simulink model "TST_InjVlv_CalcET"  (R2016b)
settings: Solver=FixedStepDiscrete  StartTime=0.0  StopTime=simTime  FixedStep=sampleTime  RelTol=1e-3
values from neighbouring files (symbols this model uses):
  testCase = 1    [initTST_InjVlv_CalcET_001.m]    (also in initTST_InjVlv_CalcET_002.m = 2)
libraries: simulink x21, UnitTest_Lib x18
settings Model: Creator=zhengjinyan  LastModifiedBy=zhengjinyan
settings DebuggingCC: SignalRangeChecking=error

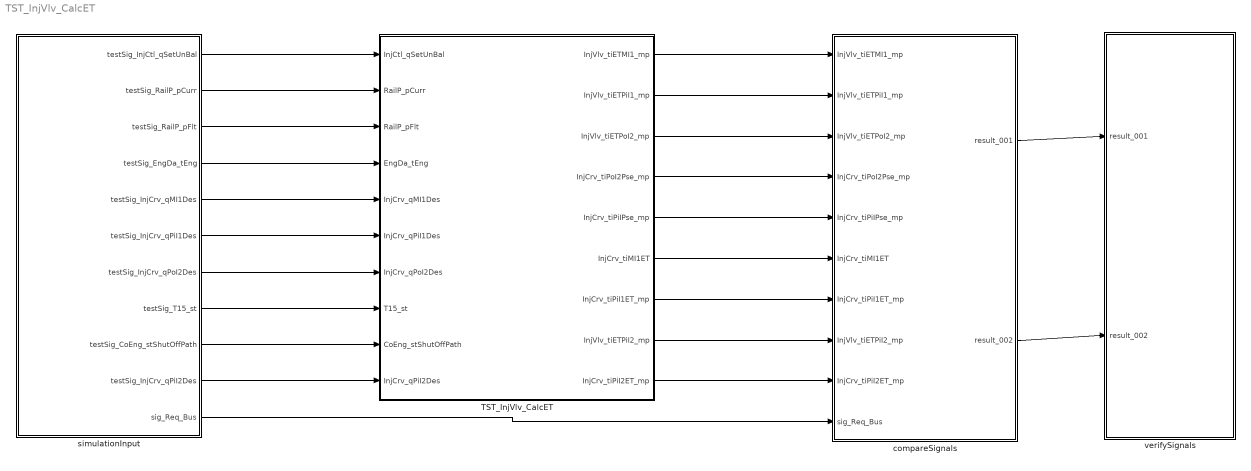
== system TST_InjVlv_CalcET ==
  TST_InjVlv_CalcET : Subsystem
  compareSignals : Subsystem
  simulationInput : Subsystem
  verifySignals : Subsystem
  wires:
  simulationInput/1(testSig_InjCtl_qSetUnBal) -> TST_InjVlv_CalcET/1(InjCtl_qSetUnBal)
  simulationInput/2(testSig_RailP_pCurr) -> TST_InjVlv_CalcET/2(RailP_pCurr)
  simulationInput/3(testSig_RailP_pFlt) -> TST_InjVlv_CalcET/3(RailP_pFlt)
  simulationInput/4(testSig_EngDa_tEng) -> TST_InjVlv_CalcET/4(EngDa_tEng)
  simulationInput/5(testSig_InjCrv_qMI1Des) -> TST_InjVlv_CalcET/5(InjCrv_qMI1Des)
  simulationInput/6(testSig_InjCrv_qPiI1Des) -> TST_InjVlv_CalcET/6(InjCrv_qPiI1Des)
  simulationInput/7(testSig_InjCrv_qPoI2Des) -> TST_InjVlv_CalcET/7(InjCrv_qPoI2Des)
  simulationInput/8(testSig_T15_st) -> TST_InjVlv_CalcET/8(T15_st)
  simulationInput/9(testSig_CoEng_stShutOffPath) -> TST_InjVlv_CalcET/9(CoEng_stShutOffPath)
  simulationInput/10(testSig_InjCrv_qPiI2Des) -> TST_InjVlv_CalcET/10(InjCrv_qPiI2Des)
  TST_InjVlv_CalcET/1(InjVlv_tiETMI1_mp) -> compareSignals/1(InjVlv_tiETMI1_mp)
  TST_InjVlv_CalcET/2(InjVlv_tiETPiI1_mp) -> compareSignals/2(InjVlv_tiETPiI1_mp)
  TST_InjVlv_CalcET/3(InjVlv_tiETPoI2_mp) -> compareSignals/3(InjVlv_tiETPoI2_mp)
  TST_InjVlv_CalcET/4(InjCrv_tiPoI2Pse_mp) -> compareSignals/4(InjCrv_tiPoI2Pse_mp)
  TST_InjVlv_CalcET/5(InjCrv_tiPiIPse_mp) -> compareSignals/5(InjCrv_tiPiIPse_mp)
  TST_InjVlv_CalcET/6(InjCrv_tiMI1ET) -> compareSignals/6(InjCrv_tiMI1ET)
  TST_InjVlv_CalcET/7(InjCrv_tiPiI1ET_mp) -> compareSignals/7(InjCrv_tiPiI1ET_mp)
  TST_InjVlv_CalcET/8(InjVlv_tiETPiI2_mp) -> compareSignals/8(InjVlv_tiETPiI2_mp)
  TST_InjVlv_CalcET/9(InjCrv_tiPiI2ET_mp) -> compareSignals/9(InjCrv_tiPiI2ET_mp)
  simulationInput/11(sig_Req_Bus) -> compareSignals/10(sig_Req_Bus)
  compareSignals/1(result_001) -> verifySignals/1(result_001)
  compareSignals/2(result_002) -> verifySignals/2(result_002)

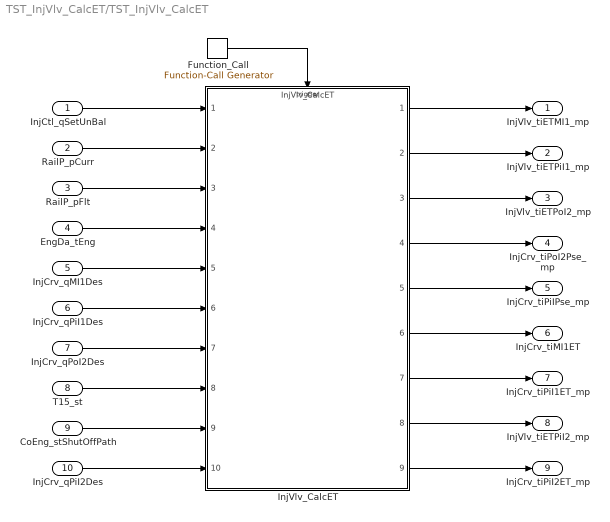
== system TST_InjVlv_CalcET/TST_InjVlv_CalcET ==
  InjCtl_qSetUnBal : Inport
  RailP_pCurr : Inport  Port=2
  RailP_pFlt : Inport  Port=3
  EngDa_tEng : Inport  Port=4
  InjCrv_qMI1Des : Inport  Port=5
  InjCrv_qPiI1Des : Inport  Port=6
  InjCrv_qPoI2Des : Inport  Port=7
  T15_st : Inport  Port=8
  CoEng_stShutOffPath : Inport  Port=9
  InjCrv_qPiI2Des : Inport  Port=10
  Function_Call : simulink/Ports & Subsystems/Function-Call Generator  sample_time=sampleTime  numberOfIterations=1
  InjVlv_CalcET : ModelReference  ModelNameDialog=InjVlv_CalcET  SimulationMode=Normal  ModelReferenceVersion=1.43  TriggerPortName=function  TriggerPortTriggerType=function-call  TriggerPortStatesWhenEnabling=held
  InjVlv_tiETMI1_mp : Outport
  InjVlv_tiETPiI1_mp : Outport  Port=2
  InjVlv_tiETPoI2_mp : Outport  Port=3
  InjCrv_tiPoI2Pse_mp : Outport  Port=4
  InjCrv_tiPiIPse_mp : Outport  Port=5
  InjCrv_tiMI1ET : Outport  Port=6
  InjCrv_tiPiI1ET_mp : Outport  Port=7
  InjVlv_tiETPiI2_mp : Outport  Port=8
  InjCrv_tiPiI2ET_mp : Outport  Port=9
  wires:
  Function_Call/1 -> InjVlv_CalcET/Trigger
  InjCtl_qSetUnBal/1 -> InjVlv_CalcET/1
  RailP_pCurr/1 -> InjVlv_CalcET/2
  RailP_pFlt/1 -> InjVlv_CalcET/3
  EngDa_tEng/1 -> InjVlv_CalcET/4
  InjCrv_qMI1Des/1 -> InjVlv_CalcET/5
  InjCrv_qPiI1Des/1 -> InjVlv_CalcET/6
  InjCrv_qPoI2Des/1 -> InjVlv_CalcET/7
  T15_st/1 -> InjVlv_CalcET/8
  CoEng_stShutOffPath/1 -> InjVlv_CalcET/9
  InjCrv_qPiI2Des/1 -> InjVlv_CalcET/10
  InjVlv_CalcET/1 -> InjVlv_tiETMI1_mp/1
  InjVlv_CalcET/2 -> InjVlv_tiETPiI1_mp/1
  InjVlv_CalcET/3 -> InjVlv_tiETPoI2_mp/1
  InjVlv_CalcET/4 -> InjCrv_tiPoI2Pse_mp/1
  InjVlv_CalcET/5 -> InjCrv_tiPiIPse_mp/1
  InjVlv_CalcET/6 -> InjCrv_tiMI1ET/1
  InjVlv_CalcET/7 -> InjCrv_tiPiI1ET_mp/1
  InjVlv_CalcET/8 -> InjVlv_tiETPiI2_mp/1
  InjVlv_CalcET/9 -> InjCrv_tiPiI2ET_mp/1

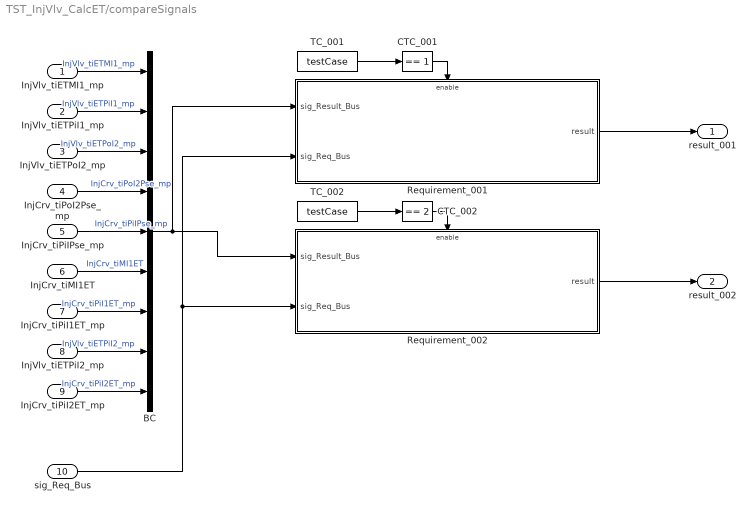
== system TST_InjVlv_CalcET/compareSignals ==
  InjVlv_tiETMI1_mp : Inport
  InjVlv_tiETPiI1_mp : Inport  Port=2
  InjVlv_tiETPoI2_mp : Inport  Port=3
  InjCrv_tiPoI2Pse_mp : Inport  Port=4
  InjCrv_tiPiIPse_mp : Inport  Port=5
  InjCrv_tiMI1ET : Inport  Port=6
  InjCrv_tiPiI1ET_mp : Inport  Port=7
  InjVlv_tiETPiI2_mp : Inport  Port=8
  InjCrv_tiPiI2ET_mp : Inport  Port=9
  sig_Req_Bus : Inport  Port=10
  BC : BusCreator  Inputs=9
  CTC_001 : simulink/Logic and Bit Operations/Compare To Constant  relop===  const=1  OutDataTypeStr=boolean
  CTC_002 : simulink/Logic and Bit Operations/Compare To Constant  relop===  const=2  OutDataTypeStr=boolean
  Requirement_001 : Subsystem
  Requirement_002 : Subsystem
  TC_001 : Constant  Value=testCase
  TC_002 : Constant  Value=testCase
  result_001 : Outport
  result_002 : Outport  Port=2
  wires:
  InjVlv_tiETMI1_mp/1 -> BC/1  "InjVlv_tiETMI1_mp"
  InjVlv_tiETPiI1_mp/1 -> BC/2  "InjVlv_tiETPiI1_mp"
  InjVlv_tiETPoI2_mp/1 -> BC/3  "InjVlv_tiETPoI2_mp"
  InjCrv_tiPoI2Pse_mp/1 -> BC/4  "InjCrv_tiPoI2Pse_mp"
  InjCrv_tiPiIPse_mp/1 -> BC/5  "InjCrv_tiPiIPse_mp"
  InjCrv_tiMI1ET/1 -> BC/6  "InjCrv_tiMI1ET"
  InjCrv_tiPiI1ET_mp/1 -> BC/7  "InjCrv_tiPiI1ET_mp"
  InjVlv_tiETPiI2_mp/1 -> BC/8  "InjVlv_tiETPiI2_mp"
  InjCrv_tiPiI2ET_mp/1 -> BC/9  "InjCrv_tiPiI2ET_mp"
  TC_001/1 -> CTC_001/1
  CTC_001/1 -> Requirement_001/Enable
  sig_Req_Bus/1 -> Requirement_001/2(sig_Req_Bus), Requirement_002/2(sig_Req_Bus)
  BC/1 -> Requirement_001/1(sig_Result_Bus), Requirement_002/1(sig_Result_Bus)
  Requirement_001/1(result) -> result_001/1
  TC_002/1 -> CTC_002/1
  CTC_002/1 -> Requirement_002/Enable
  Requirement_002/1(result) -> result_002/1

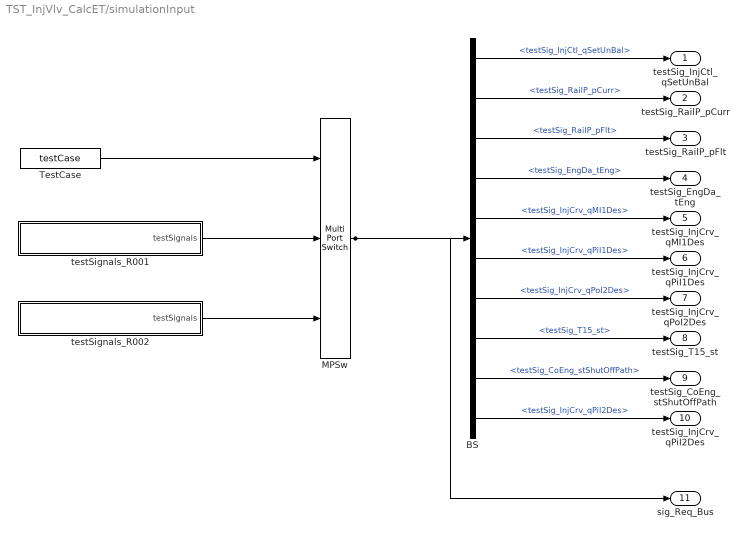
== system TST_InjVlv_CalcET/simulationInput ==
  BS : BusSelector  OutputSignals=testSig_InjCtl_qSetUnBal,testSig_RailP_pCurr,testSig_RailP_pFlt,testSig_EngDa_tEng,testSig_InjCrv_qMI1Des,testSig_InjCrv_qPiI1Des,testSig_InjCrv_qPoI2Des,testSig_T15_st,testSig_CoEng_stShutOffPath,testSig_InjCrv_qPiI2Des
  MPSw : MultiPortSwitch  Inputs=2  SaturateOnIntegerOverflow=on  InputSameDT=on
  TestCase : Constant  Value=testCase
  testSignals_R001 : Subsystem
  testSignals_R002 : Subsystem
  testSig_InjCtl_qSetUnBal : Outport
  testSig_RailP_pCurr : Outport  Port=2
  testSig_RailP_pFlt : Outport  Port=3
  testSig_EngDa_tEng : Outport  Port=4
  testSig_InjCrv_qMI1Des : Outport  Port=5
  testSig_InjCrv_qPiI1Des : Outport  Port=6
  testSig_InjCrv_qPoI2Des : Outport  Port=7
  testSig_T15_st : Outport  Port=8
  testSig_CoEng_stShutOffPath : Outport  Port=9
  testSig_InjCrv_qPiI2Des : Outport  Port=10
  sig_Req_Bus : Outport  Port=11
  wires:
  BS/1 -> testSig_InjCtl_qSetUnBal/1  "<testSig_InjCtl_qSetUnBal>"
  BS/2 -> testSig_RailP_pCurr/1  "<testSig_RailP_pCurr>"
  BS/3 -> testSig_RailP_pFlt/1  "<testSig_RailP_pFlt>"
  BS/4 -> testSig_EngDa_tEng/1  "<testSig_EngDa_tEng>"
  BS/5 -> testSig_InjCrv_qMI1Des/1  "<testSig_InjCrv_qMI1Des>"
  BS/6 -> testSig_InjCrv_qPiI1Des/1  "<testSig_InjCrv_qPiI1Des>"
  BS/7 -> testSig_InjCrv_qPoI2Des/1  "<testSig_InjCrv_qPoI2Des>"
  BS/8 -> testSig_T15_st/1  "<testSig_T15_st>"
  BS/9 -> testSig_CoEng_stShutOffPath/1  "<testSig_CoEng_stShutOffPath>"
  BS/10 -> testSig_InjCrv_qPiI2Des/1  "<testSig_InjCrv_qPiI2Des>"
  MPSw/1 -> BS/1, sig_Req_Bus/1
  TestCase/1 -> MPSw/1
  testSignals_R001/1(testSignals) -> MPSw/2
  testSignals_R002/1(testSignals) -> MPSw/3

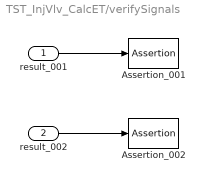
== system TST_InjVlv_CalcET/verifySignals ==
  result_001 : Inport
  result_002 : Inport  Port=2
  Assertion_001 : Assertion  Enabled=off
  Assertion_002 : Assertion  Enabled=off
  wires:
  result_001/1 -> Assertion_001/1
  result_002/1 -> Assertion_002/1

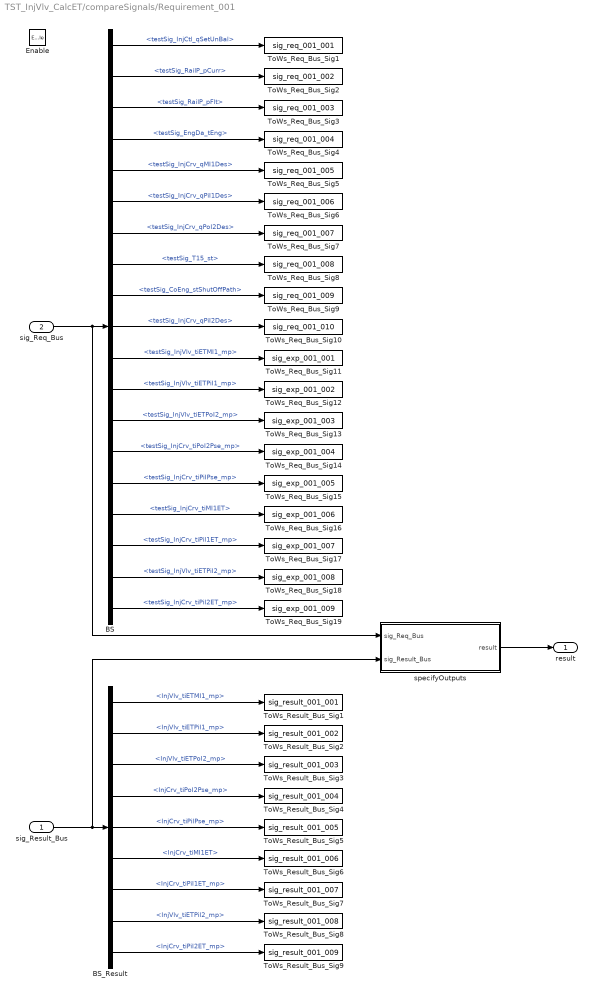
== system TST_InjVlv_CalcET/compareSignals/Requirement_001 ==
  sig_Result_Bus : Inport
  sig_Req_Bus : Inport  Port=2
  Enable : EnablePort
  BS : BusSelector  OutputSignals=testSig_InjCtl_qSetUnBal,testSig_RailP_pCurr,testSig_RailP_pFlt,testSig_EngDa_tEng,testSig_InjCrv_qMI1Des,testSig_InjCrv_qPiI1Des,testSig_InjCrv_qPoI2Des,testSig_T15_st,testSig_CoEng_stShutOffPath,testSig_InjCrv_qPiI2Des,testSig_InjVlv_tiETMI1_mp,testSig_InjVlv_tiETPiI1_mp,testSig_InjVlv_tiETPoI2_mp,testSig_InjCrv_tiPoI2Pse_mp,testSig_InjCrv_tiPiIPse_mp,testSig_InjCrv_tiMI1ET,testSig_InjCrv_tiPiI1ET_mp,testSig_InjVlv_tiETPiI2_mp,testSig_InjCrv_tiPiI2ET_mp
  BS_Result : BusSelector  OutputSignals=InjVlv_tiETMI1_mp,InjVlv_tiETPiI1_mp,InjVlv_tiETPoI2_mp,InjCrv_tiPoI2Pse_mp,InjCrv_tiPiIPse_mp,InjCrv_tiMI1ET,InjCrv_tiPiI1ET_mp,InjVlv_tiETPiI2_mp,InjCrv_tiPiI2ET_mp
  ToWs_Req_Bus_Sig1 : ToWorkspace  VariableName=sig_req_001_001  SaveFormat=Structure With Time
  ToWs_Req_Bus_Sig10 : ToWorkspace  VariableName=sig_req_001_010  SaveFormat=Structure With Time
  ToWs_Req_Bus_Sig11 : ToWorkspace  VariableName=sig_exp_001_001  SaveFormat=Structure With Time
  ToWs_Req_Bus_Sig12 : ToWorkspace  VariableName=sig_exp_001_002  SaveFormat=Structure With Time
  ToWs_Req_Bus_Sig13 : ToWorkspace  VariableName=sig_exp_001_003  SaveFormat=Structure With Time
  ToWs_Req_Bus_Sig14 : ToWorkspace  VariableName=sig_exp_001_004  SaveFormat=Structure With Time
  ToWs_Req_Bus_Sig15 : ToWorkspace  VariableName=sig_exp_001_005  SaveFormat=Structure With Time
  ToWs_Req_Bus_Sig16 : ToWorkspace  VariableName=sig_exp_001_006  SaveFormat=Structure With Time
  ToWs_Req_Bus_Sig17 : ToWorkspace  VariableName=sig_exp_001_007  SaveFormat=Structure With Time
  ToWs_Req_Bus_Sig18 : ToWorkspace  VariableName=sig_exp_001_008  SaveFormat=Structure With Time
  ToWs_Req_Bus_Sig19 : ToWorkspace  VariableName=sig_exp_001_009  SaveFormat=Structure With Time
  ToWs_Req_Bus_Sig2 : ToWorkspace  VariableName=sig_req_001_002  SaveFormat=Structure With Time
  ToWs_Req_Bus_Sig3 : ToWorkspace  VariableName=sig_req_001_003  SaveFormat=Structure With Time
  ToWs_Req_Bus_Sig4 : ToWorkspace  VariableName=sig_req_001_004  SaveFormat=Structure With Time
  ToWs_Req_Bus_Sig5 : ToWorkspace  VariableName=sig_req_001_005  SaveFormat=Structure With Time
  ToWs_Req_Bus_Sig6 : ToWorkspace  VariableName=sig_req_001_006  SaveFormat=Structure With Time
  ToWs_Req_Bus_Sig7 : ToWorkspace  VariableName=sig_req_001_007  SaveFormat=Structure With Time
  ToWs_Req_Bus_Sig8 : ToWorkspace  VariableName=sig_req_001_008  SaveFormat=Structure With Time
  ToWs_Req_Bus_Sig9 : ToWorkspace  VariableName=sig_req_001_009  SaveFormat=Structure With Time
  ToWs_Result_Bus_Sig1 : ToWorkspace  VariableName=sig_result_001_001  SaveFormat=Structure With Time
  ToWs_Result_Bus_Sig2 : ToWorkspace  VariableName=sig_result_001_002  SaveFormat=Structure With Time
  ToWs_Result_Bus_Sig3 : ToWorkspace  VariableName=sig_result_001_003  SaveFormat=Structure With Time
  ToWs_Result_Bus_Sig4 : ToWorkspace  VariableName=sig_result_001_004  SaveFormat=Structure With Time
  ToWs_Result_Bus_Sig5 : ToWorkspace  VariableName=sig_result_001_005  SaveFormat=Structure With Time
  ToWs_Result_Bus_Sig6 : ToWorkspace  VariableName=sig_result_001_006  SaveFormat=Structure With Time
  ToWs_Result_Bus_Sig7 : ToWorkspace  VariableName=sig_result_001_007  SaveFormat=Structure With Time
  ToWs_Result_Bus_Sig8 : ToWorkspace  VariableName=sig_result_001_008  SaveFormat=Structure With Time
  ToWs_Result_Bus_Sig9 : ToWorkspace  VariableName=sig_result_001_009  SaveFormat=Structure With Time
  specifyOutputs : Subsystem
  result : Outport
  wires:
  sig_Req_Bus/1 -> BS/1, specifyOutputs/1(sig_Req_Bus)
  BS/1 -> ToWs_Req_Bus_Sig1/1  "<testSig_InjCtl_qSetUnBal>"
  BS/2 -> ToWs_Req_Bus_Sig2/1  "<testSig_RailP_pCurr>"
  BS/3 -> ToWs_Req_Bus_Sig3/1  "<testSig_RailP_pFlt>"
  BS/4 -> ToWs_Req_Bus_Sig4/1  "<testSig_EngDa_tEng>"
  BS/5 -> ToWs_Req_Bus_Sig5/1  "<testSig_InjCrv_qMI1Des>"
  BS/6 -> ToWs_Req_Bus_Sig6/1  "<testSig_InjCrv_qPiI1Des>"
  BS/7 -> ToWs_Req_Bus_Sig7/1  "<testSig_InjCrv_qPoI2Des>"
  BS/8 -> ToWs_Req_Bus_Sig8/1  "<testSig_T15_st>"
  BS/9 -> ToWs_Req_Bus_Sig9/1  "<testSig_CoEng_stShutOffPath>"
  BS/10 -> ToWs_Req_Bus_Sig10/1  "<testSig_InjCrv_qPiI2Des>"
  BS/11 -> ToWs_Req_Bus_Sig11/1  "<testSig_InjVlv_tiETMI1_mp>"
  BS/12 -> ToWs_Req_Bus_Sig12/1  "<testSig_InjVlv_tiETPiI1_mp>"
  BS/13 -> ToWs_Req_Bus_Sig13/1  "<testSig_InjVlv_tiETPoI2_mp>"
  BS/14 -> ToWs_Req_Bus_Sig14/1  "<testSig_InjCrv_tiPoI2Pse_mp>"
  BS/15 -> ToWs_Req_Bus_Sig15/1  "<testSig_InjCrv_tiPiIPse_mp>"
  BS/16 -> ToWs_Req_Bus_Sig16/1  "<testSig_InjCrv_tiMI1ET>"
  BS/17 -> ToWs_Req_Bus_Sig17/1  "<testSig_InjCrv_tiPiI1ET_mp>"
  BS/18 -> ToWs_Req_Bus_Sig18/1  "<testSig_InjVlv_tiETPiI2_mp>"
  BS/19 -> ToWs_Req_Bus_Sig19/1  "<testSig_InjCrv_tiPiI2ET_mp>"
  sig_Result_Bus/1 -> BS_Result/1, specifyOutputs/2(sig_Result_Bus)
  BS_Result/1 -> ToWs_Result_Bus_Sig1/1  "<InjVlv_tiETMI1_mp>"
  BS_Result/2 -> ToWs_Result_Bus_Sig2/1  "<InjVlv_tiETPiI1_mp>"
  BS_Result/3 -> ToWs_Result_Bus_Sig3/1  "<InjVlv_tiETPoI2_mp>"
  BS_Result/4 -> ToWs_Result_Bus_Sig4/1  "<InjCrv_tiPoI2Pse_mp>"
  BS_Result/5 -> ToWs_Result_Bus_Sig5/1  "<InjCrv_tiPiIPse_mp>"
  BS_Result/6 -> ToWs_Result_Bus_Sig6/1  "<InjCrv_tiMI1ET>"
  BS_Result/7 -> ToWs_Result_Bus_Sig7/1  "<InjCrv_tiPiI1ET_mp>"
  BS_Result/8 -> ToWs_Result_Bus_Sig8/1  "<InjVlv_tiETPiI2_mp>"
  BS_Result/9 -> ToWs_Result_Bus_Sig9/1  "<InjCrv_tiPiI2ET_mp>"
  specifyOutputs/1(result) -> result/1

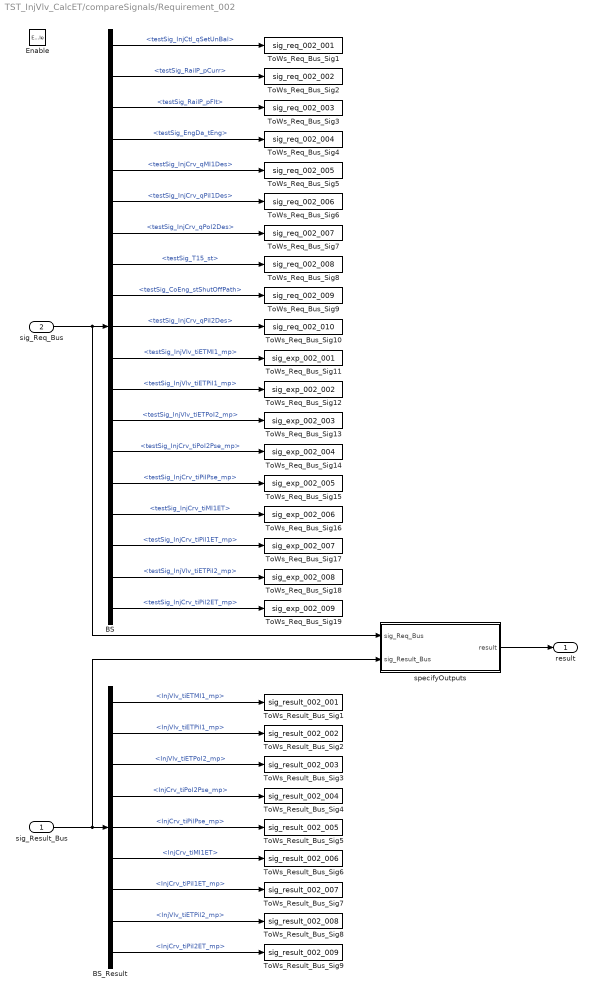
== system TST_InjVlv_CalcET/compareSignals/Requirement_002 ==
  sig_Result_Bus : Inport
  sig_Req_Bus : Inport  Port=2
  Enable : EnablePort
  BS : BusSelector  OutputSignals=testSig_InjCtl_qSetUnBal,testSig_RailP_pCurr,testSig_RailP_pFlt,testSig_EngDa_tEng,testSig_InjCrv_qMI1Des,testSig_InjCrv_qPiI1Des,testSig_InjCrv_qPoI2Des,testSig_T15_st,testSig_CoEng_stShutOffPath,testSig_InjCrv_qPiI2Des,testSig_InjVlv_tiETMI1_mp,testSig_InjVlv_tiETPiI1_mp,testSig_InjVlv_tiETPoI2_mp,testSig_InjCrv_tiPoI2Pse_mp,testSig_InjCrv_tiPiIPse_mp,testSig_InjCrv_tiMI1ET,testSig_InjCrv_tiPiI1ET_mp,testSig_InjVlv_tiETPiI2_mp,testSig_InjCrv_tiPiI2ET_mp
  BS_Result : BusSelector  OutputSignals=InjVlv_tiETMI1_mp,InjVlv_tiETPiI1_mp,InjVlv_tiETPoI2_mp,InjCrv_tiPoI2Pse_mp,InjCrv_tiPiIPse_mp,InjCrv_tiMI1ET,InjCrv_tiPiI1ET_mp,InjVlv_tiETPiI2_mp,InjCrv_tiPiI2ET_mp
  ToWs_Req_Bus_Sig1 : ToWorkspace  VariableName=sig_req_002_001  SaveFormat=Structure With Time
  ToWs_Req_Bus_Sig10 : ToWorkspace  VariableName=sig_req_002_010  SaveFormat=Structure With Time
  ToWs_Req_Bus_Sig11 : ToWorkspace  VariableName=sig_exp_002_001  SaveFormat=Structure With Time
  ToWs_Req_Bus_Sig12 : ToWorkspace  VariableName=sig_exp_002_002  SaveFormat=Structure With Time
  ToWs_Req_Bus_Sig13 : ToWorkspace  VariableName=sig_exp_002_003  SaveFormat=Structure With Time
  ToWs_Req_Bus_Sig14 : ToWorkspace  VariableName=sig_exp_002_004  SaveFormat=Structure With Time
  ToWs_Req_Bus_Sig15 : ToWorkspace  VariableName=sig_exp_002_005  SaveFormat=Structure With Time
  ToWs_Req_Bus_Sig16 : ToWorkspace  VariableName=sig_exp_002_006  SaveFormat=Structure With Time
  ToWs_Req_Bus_Sig17 : ToWorkspace  VariableName=sig_exp_002_007  SaveFormat=Structure With Time
  ToWs_Req_Bus_Sig18 : ToWorkspace  VariableName=sig_exp_002_008  SaveFormat=Structure With Time
  ToWs_Req_Bus_Sig19 : ToWorkspace  VariableName=sig_exp_002_009  SaveFormat=Structure With Time
  ToWs_Req_Bus_Sig2 : ToWorkspace  VariableName=sig_req_002_002  SaveFormat=Structure With Time
  ToWs_Req_Bus_Sig3 : ToWorkspace  VariableName=sig_req_002_003  SaveFormat=Structure With Time
  ToWs_Req_Bus_Sig4 : ToWorkspace  VariableName=sig_req_002_004  SaveFormat=Structure With Time
  ToWs_Req_Bus_Sig5 : ToWorkspace  VariableName=sig_req_002_005  SaveFormat=Structure With Time
  ToWs_Req_Bus_Sig6 : ToWorkspace  VariableName=sig_req_002_006  SaveFormat=Structure With Time
  ToWs_Req_Bus_Sig7 : ToWorkspace  VariableName=sig_req_002_007  SaveFormat=Structure With Time
  ToWs_Req_Bus_Sig8 : ToWorkspace  VariableName=sig_req_002_008  SaveFormat=Structure With Time
  ToWs_Req_Bus_Sig9 : ToWorkspace  VariableName=sig_req_002_009  SaveFormat=Structure With Time
  ToWs_Result_Bus_Sig1 : ToWorkspace  VariableName=sig_result_002_001  SaveFormat=Structure With Time
  ToWs_Result_Bus_Sig2 : ToWorkspace  VariableName=sig_result_002_002  SaveFormat=Structure With Time
  ToWs_Result_Bus_Sig3 : ToWorkspace  VariableName=sig_result_002_003  SaveFormat=Structure With Time
  ToWs_Result_Bus_Sig4 : ToWorkspace  VariableName=sig_result_002_004  SaveFormat=Structure With Time
  ToWs_Result_Bus_Sig5 : ToWorkspace  VariableName=sig_result_002_005  SaveFormat=Structure With Time
  ToWs_Result_Bus_Sig6 : ToWorkspace  VariableName=sig_result_002_006  SaveFormat=Structure With Time
  ToWs_Result_Bus_Sig7 : ToWorkspace  VariableName=sig_result_002_007  SaveFormat=Structure With Time
  ToWs_Result_Bus_Sig8 : ToWorkspace  VariableName=sig_result_002_008  SaveFormat=Structure With Time
  ToWs_Result_Bus_Sig9 : ToWorkspace  VariableName=sig_result_002_009  SaveFormat=Structure With Time
  specifyOutputs : Subsystem
  result : Outport
  wires:
  sig_Req_Bus/1 -> BS/1, specifyOutputs/1(sig_Req_Bus)
  BS/1 -> ToWs_Req_Bus_Sig1/1  "<testSig_InjCtl_qSetUnBal>"
  BS/2 -> ToWs_Req_Bus_Sig2/1  "<testSig_RailP_pCurr>"
  BS/3 -> ToWs_Req_Bus_Sig3/1  "<testSig_RailP_pFlt>"
  BS/4 -> ToWs_Req_Bus_Sig4/1  "<testSig_EngDa_tEng>"
  BS/5 -> ToWs_Req_Bus_Sig5/1  "<testSig_InjCrv_qMI1Des>"
  BS/6 -> ToWs_Req_Bus_Sig6/1  "<testSig_InjCrv_qPiI1Des>"
  BS/7 -> ToWs_Req_Bus_Sig7/1  "<testSig_InjCrv_qPoI2Des>"
  BS/8 -> ToWs_Req_Bus_Sig8/1  "<testSig_T15_st>"
  BS/9 -> ToWs_Req_Bus_Sig9/1  "<testSig_CoEng_stShutOffPath>"
  BS/10 -> ToWs_Req_Bus_Sig10/1  "<testSig_InjCrv_qPiI2Des>"
  BS/11 -> ToWs_Req_Bus_Sig11/1  "<testSig_InjVlv_tiETMI1_mp>"
  BS/12 -> ToWs_Req_Bus_Sig12/1  "<testSig_InjVlv_tiETPiI1_mp>"
  BS/13 -> ToWs_Req_Bus_Sig13/1  "<testSig_InjVlv_tiETPoI2_mp>"
  BS/14 -> ToWs_Req_Bus_Sig14/1  "<testSig_InjCrv_tiPoI2Pse_mp>"
  BS/15 -> ToWs_Req_Bus_Sig15/1  "<testSig_InjCrv_tiPiIPse_mp>"
  BS/16 -> ToWs_Req_Bus_Sig16/1  "<testSig_InjCrv_tiMI1ET>"
  BS/17 -> ToWs_Req_Bus_Sig17/1  "<testSig_InjCrv_tiPiI1ET_mp>"
  BS/18 -> ToWs_Req_Bus_Sig18/1  "<testSig_InjVlv_tiETPiI2_mp>"
  BS/19 -> ToWs_Req_Bus_Sig19/1  "<testSig_InjCrv_tiPiI2ET_mp>"
  sig_Result_Bus/1 -> BS_Result/1, specifyOutputs/2(sig_Result_Bus)
  BS_Result/1 -> ToWs_Result_Bus_Sig1/1  "<InjVlv_tiETMI1_mp>"
  BS_Result/2 -> ToWs_Result_Bus_Sig2/1  "<InjVlv_tiETPiI1_mp>"
  BS_Result/3 -> ToWs_Result_Bus_Sig3/1  "<InjVlv_tiETPoI2_mp>"
  BS_Result/4 -> ToWs_Result_Bus_Sig4/1  "<InjCrv_tiPoI2Pse_mp>"
  BS_Result/5 -> ToWs_Result_Bus_Sig5/1  "<InjCrv_tiPiIPse_mp>"
  BS_Result/6 -> ToWs_Result_Bus_Sig6/1  "<InjCrv_tiMI1ET>"
  BS_Result/7 -> ToWs_Result_Bus_Sig7/1  "<InjCrv_tiPiI1ET_mp>"
  BS_Result/8 -> ToWs_Result_Bus_Sig8/1  "<InjVlv_tiETPiI2_mp>"
  BS_Result/9 -> ToWs_Result_Bus_Sig9/1  "<InjCrv_tiPiI2ET_mp>"
  specifyOutputs/1(result) -> result/1

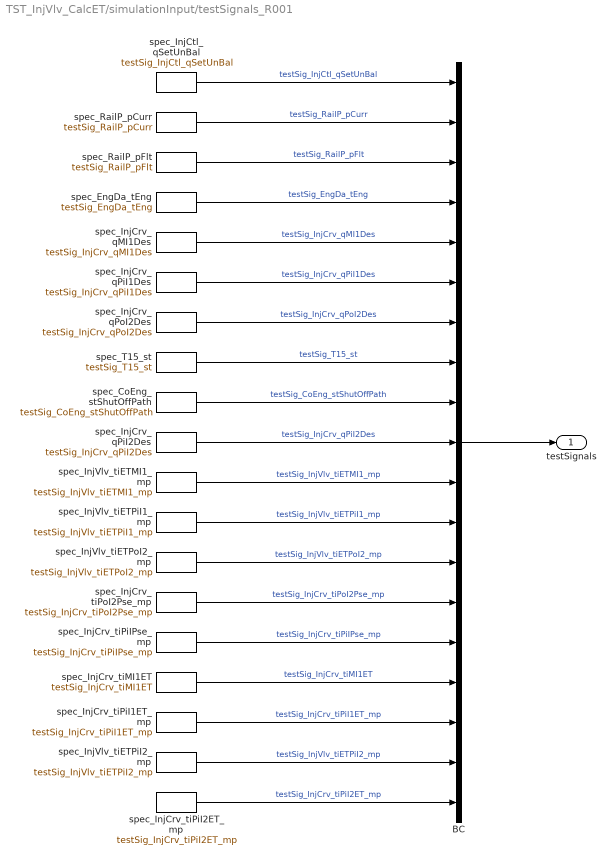
== system TST_InjVlv_CalcET/simulationInput/testSignals_R001 ==
  BC : BusCreator  Inputs=19
  spec_CoEng_stShutOffPath : FromWorkspace  VariableName=testSig_CoEng_stShutOffPath  Interpolate=off  OutputAfterFinalValue=Holding final value
  spec_EngDa_tEng : FromWorkspace  VariableName=testSig_EngDa_tEng  Interpolate=off  OutputAfterFinalValue=Holding final value
  spec_InjCrv_qMI1Des : FromWorkspace  VariableName=testSig_InjCrv_qMI1Des  Interpolate=off  OutputAfterFinalValue=Holding final value
  spec_InjCrv_qPiI1Des : FromWorkspace  VariableName=testSig_InjCrv_qPiI1Des  Interpolate=off  OutputAfterFinalValue=Holding final value
  spec_InjCrv_qPiI2Des : FromWorkspace  VariableName=testSig_InjCrv_qPiI2Des  Interpolate=off  OutputAfterFinalValue=Holding final value
  spec_InjCrv_qPoI2Des : FromWorkspace  VariableName=testSig_InjCrv_qPoI2Des  Interpolate=off  OutputAfterFinalValue=Holding final value
  spec_InjCrv_tiMI1ET : FromWorkspace  VariableName=testSig_InjCrv_tiMI1ET  Interpolate=off  OutputAfterFinalValue=Holding final value
  spec_InjCrv_tiPiI1ET_mp : FromWorkspace  VariableName=testSig_InjCrv_tiPiI1ET_mp  Interpolate=off  OutputAfterFinalValue=Holding final value
  spec_InjCrv_tiPiI2ET_mp : FromWorkspace  VariableName=testSig_InjCrv_tiPiI2ET_mp  Interpolate=off  OutputAfterFinalValue=Holding final value
  spec_InjCrv_tiPiIPse_mp : FromWorkspace  VariableName=testSig_InjCrv_tiPiIPse_mp  Interpolate=off  OutputAfterFinalValue=Holding final value
  spec_InjCrv_tiPoI2Pse_mp : FromWorkspace  VariableName=testSig_InjCrv_tiPoI2Pse_mp  Interpolate=off  OutputAfterFinalValue=Holding final value
  spec_InjCtl_qSetUnBal : FromWorkspace  VariableName=testSig_InjCtl_qSetUnBal  Interpolate=off  OutputAfterFinalValue=Holding final value
  spec_InjVlv_tiETMI1_mp : FromWorkspace  VariableName=testSig_InjVlv_tiETMI1_mp  Interpolate=off  OutputAfterFinalValue=Holding final value
  spec_InjVlv_tiETPiI1_mp : FromWorkspace  VariableName=testSig_InjVlv_tiETPiI1_mp  Interpolate=off  OutputAfterFinalValue=Holding final value
  spec_InjVlv_tiETPiI2_mp : FromWorkspace  VariableName=testSig_InjVlv_tiETPiI2_mp  Interpolate=off  OutputAfterFinalValue=Holding final value
  spec_InjVlv_tiETPoI2_mp : FromWorkspace  VariableName=testSig_InjVlv_tiETPoI2_mp  Interpolate=off  OutputAfterFinalValue=Holding final value
  spec_RailP_pCurr : FromWorkspace  VariableName=testSig_RailP_pCurr  Interpolate=off  OutputAfterFinalValue=Holding final value
  spec_RailP_pFlt : FromWorkspace  VariableName=testSig_RailP_pFlt  Interpolate=off  OutputAfterFinalValue=Holding final value
  spec_T15_st : FromWorkspace  VariableName=testSig_T15_st  Interpolate=off  OutputAfterFinalValue=Holding final value
  testSignals : Outport
  wires:
  BC/1 -> testSignals/1
  spec_InjCtl_qSetUnBal/1 -> BC/1  "testSig_InjCtl_qSetUnBal"
  spec_RailP_pCurr/1 -> BC/2  "testSig_RailP_pCurr"
  spec_RailP_pFlt/1 -> BC/3  "testSig_RailP_pFlt"
  spec_EngDa_tEng/1 -> BC/4  "testSig_EngDa_tEng"
  spec_InjCrv_qMI1Des/1 -> BC/5  "testSig_InjCrv_qMI1Des"
  spec_InjCrv_qPiI1Des/1 -> BC/6  "testSig_InjCrv_qPiI1Des"
  spec_InjCrv_qPoI2Des/1 -> BC/7  "testSig_InjCrv_qPoI2Des"
  spec_T15_st/1 -> BC/8  "testSig_T15_st"
  spec_CoEng_stShutOffPath/1 -> BC/9  "testSig_CoEng_stShutOffPath"
  spec_InjCrv_qPiI2Des/1 -> BC/10  "testSig_InjCrv_qPiI2Des"
  spec_InjVlv_tiETMI1_mp/1 -> BC/11  "testSig_InjVlv_tiETMI1_mp"
  spec_InjVlv_tiETPiI1_mp/1 -> BC/12  "testSig_InjVlv_tiETPiI1_mp"
  spec_InjVlv_tiETPoI2_mp/1 -> BC/13  "testSig_InjVlv_tiETPoI2_mp"
  spec_InjCrv_tiPoI2Pse_mp/1 -> BC/14  "testSig_InjCrv_tiPoI2Pse_mp"
  spec_InjCrv_tiPiIPse_mp/1 -> BC/15  "testSig_InjCrv_tiPiIPse_mp"
  spec_InjCrv_tiMI1ET/1 -> BC/16  "testSig_InjCrv_tiMI1ET"
  spec_InjCrv_tiPiI1ET_mp/1 -> BC/17  "testSig_InjCrv_tiPiI1ET_mp"
  spec_InjVlv_tiETPiI2_mp/1 -> BC/18  "testSig_InjVlv_tiETPiI2_mp"
  spec_InjCrv_tiPiI2ET_mp/1 -> BC/19  "testSig_InjCrv_tiPiI2ET_mp"

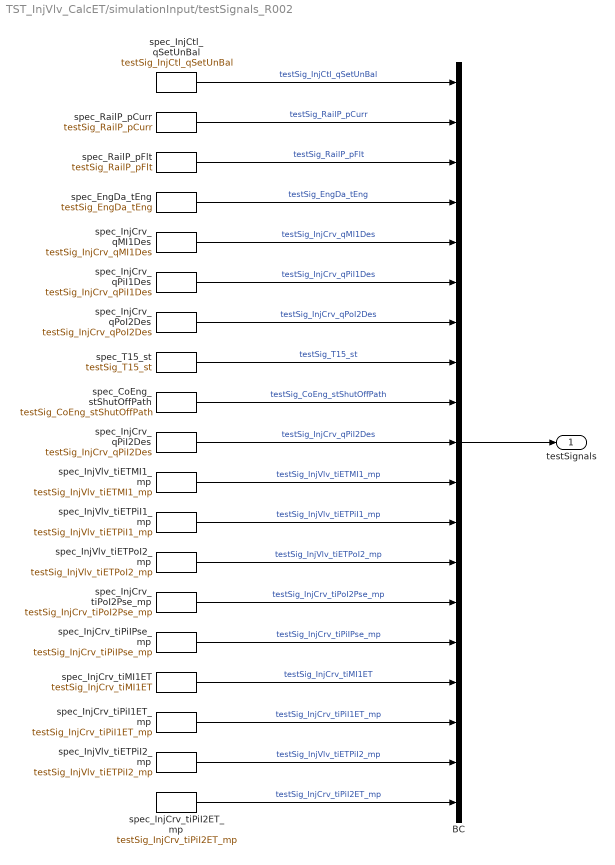
== system TST_InjVlv_CalcET/simulationInput/testSignals_R002 ==
  BC : BusCreator  Inputs=19
  spec_CoEng_stShutOffPath : FromWorkspace  VariableName=testSig_CoEng_stShutOffPath  Interpolate=off  OutputAfterFinalValue=Holding final value
  spec_EngDa_tEng : FromWorkspace  VariableName=testSig_EngDa_tEng  Interpolate=off  OutputAfterFinalValue=Holding final value
  spec_InjCrv_qMI1Des : FromWorkspace  VariableName=testSig_InjCrv_qMI1Des  Interpolate=off  OutputAfterFinalValue=Holding final value
  spec_InjCrv_qPiI1Des : FromWorkspace  VariableName=testSig_InjCrv_qPiI1Des  Interpolate=off  OutputAfterFinalValue=Holding final value
  spec_InjCrv_qPiI2Des : FromWorkspace  VariableName=testSig_InjCrv_qPiI2Des  Interpolate=off  OutputAfterFinalValue=Holding final value
  spec_InjCrv_qPoI2Des : FromWorkspace  VariableName=testSig_InjCrv_qPoI2Des  Interpolate=off  OutputAfterFinalValue=Holding final value
  spec_InjCrv_tiMI1ET : FromWorkspace  VariableName=testSig_InjCrv_tiMI1ET  Interpolate=off  OutputAfterFinalValue=Holding final value
  spec_InjCrv_tiPiI1ET_mp : FromWorkspace  VariableName=testSig_InjCrv_tiPiI1ET_mp  Interpolate=off  OutputAfterFinalValue=Holding final value
  spec_InjCrv_tiPiI2ET_mp : FromWorkspace  VariableName=testSig_InjCrv_tiPiI2ET_mp  Interpolate=off  OutputAfterFinalValue=Holding final value
  spec_InjCrv_tiPiIPse_mp : FromWorkspace  VariableName=testSig_InjCrv_tiPiIPse_mp  Interpolate=off  OutputAfterFinalValue=Holding final value
  spec_InjCrv_tiPoI2Pse_mp : FromWorkspace  VariableName=testSig_InjCrv_tiPoI2Pse_mp  Interpolate=off  OutputAfterFinalValue=Holding final value
  spec_InjCtl_qSetUnBal : FromWorkspace  VariableName=testSig_InjCtl_qSetUnBal  Interpolate=off  OutputAfterFinalValue=Holding final value
  spec_InjVlv_tiETMI1_mp : FromWorkspace  VariableName=testSig_InjVlv_tiETMI1_mp  Interpolate=off  OutputAfterFinalValue=Holding final value
  spec_InjVlv_tiETPiI1_mp : FromWorkspace  VariableName=testSig_InjVlv_tiETPiI1_mp  Interpolate=off  OutputAfterFinalValue=Holding final value
  spec_InjVlv_tiETPiI2_mp : FromWorkspace  VariableName=testSig_InjVlv_tiETPiI2_mp  Interpolate=off  OutputAfterFinalValue=Holding final value
  spec_InjVlv_tiETPoI2_mp : FromWorkspace  VariableName=testSig_InjVlv_tiETPoI2_mp  Interpolate=off  OutputAfterFinalValue=Holding final value
  spec_RailP_pCurr : FromWorkspace  VariableName=testSig_RailP_pCurr  Interpolate=off  OutputAfterFinalValue=Holding final value
  spec_RailP_pFlt : FromWorkspace  VariableName=testSig_RailP_pFlt  Interpolate=off  OutputAfterFinalValue=Holding final value
  spec_T15_st : FromWorkspace  VariableName=testSig_T15_st  Interpolate=off  OutputAfterFinalValue=Holding final value
  testSignals : Outport
  wires:
  BC/1 -> testSignals/1
  spec_InjCtl_qSetUnBal/1 -> BC/1  "testSig_InjCtl_qSetUnBal"
  spec_RailP_pCurr/1 -> BC/2  "testSig_RailP_pCurr"
  spec_RailP_pFlt/1 -> BC/3  "testSig_RailP_pFlt"
  spec_EngDa_tEng/1 -> BC/4  "testSig_EngDa_tEng"
  spec_InjCrv_qMI1Des/1 -> BC/5  "testSig_InjCrv_qMI1Des"
  spec_InjCrv_qPiI1Des/1 -> BC/6  "testSig_InjCrv_qPiI1Des"
  spec_InjCrv_qPoI2Des/1 -> BC/7  "testSig_InjCrv_qPoI2Des"
  spec_T15_st/1 -> BC/8  "testSig_T15_st"
  spec_CoEng_stShutOffPath/1 -> BC/9  "testSig_CoEng_stShutOffPath"
  spec_InjCrv_qPiI2Des/1 -> BC/10  "testSig_InjCrv_qPiI2Des"
  spec_InjVlv_tiETMI1_mp/1 -> BC/11  "testSig_InjVlv_tiETMI1_mp"
  spec_InjVlv_tiETPiI1_mp/1 -> BC/12  "testSig_InjVlv_tiETPiI1_mp"
  spec_InjVlv_tiETPoI2_mp/1 -> BC/13  "testSig_InjVlv_tiETPoI2_mp"
  spec_InjCrv_tiPoI2Pse_mp/1 -> BC/14  "testSig_InjCrv_tiPoI2Pse_mp"
  spec_InjCrv_tiPiIPse_mp/1 -> BC/15  "testSig_InjCrv_tiPiIPse_mp"
  spec_InjCrv_tiMI1ET/1 -> BC/16  "testSig_InjCrv_tiMI1ET"
  spec_InjCrv_tiPiI1ET_mp/1 -> BC/17  "testSig_InjCrv_tiPiI1ET_mp"
  spec_InjVlv_tiETPiI2_mp/1 -> BC/18  "testSig_InjVlv_tiETPiI2_mp"
  spec_InjCrv_tiPiI2ET_mp/1 -> BC/19  "testSig_InjCrv_tiPiI2ET_mp"

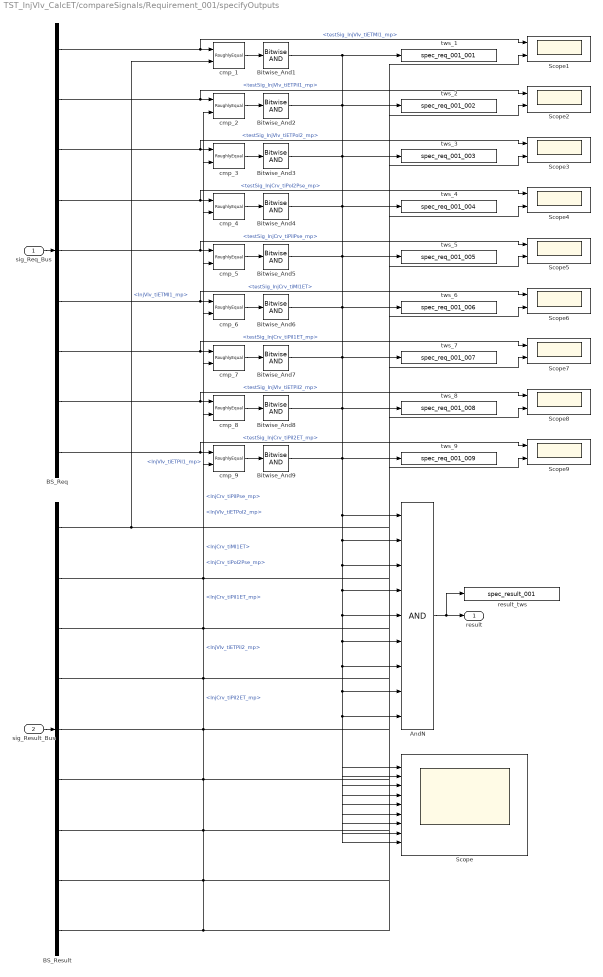
== system TST_InjVlv_CalcET/compareSignals/Requirement_001/specifyOutputs ==
  sig_Req_Bus : Inport
  sig_Result_Bus : Inport  Port=2
  AndN : Logic  Inputs=9
  BS_Req : BusSelector  OutputSignals=testSig_InjVlv_tiETMI1_mp,testSig_InjVlv_tiETPiI1_mp,testSig_InjVlv_tiETPoI2_mp,testSig_InjCrv_tiPoI2Pse_mp,testSig_InjCrv_tiPiIPse_mp,testSig_InjCrv_tiMI1ET,testSig_InjCrv_tiPiI1ET_mp,testSig_InjVlv_tiETPiI2_mp,testSig_InjCrv_tiPiI2ET_mp
  BS_Result : BusSelector  OutputSignals=InjVlv_tiETMI1_mp,InjVlv_tiETPiI1_mp,InjVlv_tiETPoI2_mp,InjCrv_tiPoI2Pse_mp,InjCrv_tiPiIPse_mp,InjCrv_tiMI1ET,InjCrv_tiPiI1ET_mp,InjVlv_tiETPiI2_mp,InjCrv_tiPiI2ET_mp
  Bitwise_And{1..9} (9 alike) : simulink/Logic and Bit Operations/Bitwise Operator  logicop=AND  UseBitMask=off  BitMask=bin2dec('11011001')  BitMaskRealWorld=Stored Integer
  Scope : Scope  NumInputPorts=9
  Scope{1..9} (9 alike) : Scope  NumInputPorts=2
  cmp_{1..9} (9 alike) : UnitTest_Lib/RoughlyEqual  slope=1
  result_tws : ToWorkspace  VariableName=spec_result_001
  tws_1 : ToWorkspace  VariableName=spec_req_001_001
  tws_2 : ToWorkspace  VariableName=spec_req_001_002
  tws_3 : ToWorkspace  VariableName=spec_req_001_003
  tws_4 : ToWorkspace  VariableName=spec_req_001_004
  tws_5 : ToWorkspace  VariableName=spec_req_001_005
  tws_6 : ToWorkspace  VariableName=spec_req_001_006
  tws_7 : ToWorkspace  VariableName=spec_req_001_007
  tws_8 : ToWorkspace  VariableName=spec_req_001_008
  tws_9 : ToWorkspace  VariableName=spec_req_001_009
  result : Outport
  wires:
  sig_Req_Bus/1 -> BS_Req/1
  sig_Result_Bus/1 -> BS_Result/1
  AndN/1 -> result/1, result_tws/1
  BS_Req/1 -> cmp_1/1, Scope1/1  "<testSig_InjVlv_tiETMI1_mp>"
  BS_Result/1 -> cmp_1/2, Scope1/2  "<InjVlv_tiETMI1_mp>"
  cmp_1/1 -> Bitwise_And1/1
  Bitwise_And1/1 -> AndN/1, Scope/1, tws_1/1
  BS_Req/2 -> cmp_2/1, Scope2/1  "<testSig_InjVlv_tiETPiI1_mp>"
  BS_Result/2 -> cmp_2/2, Scope2/2  "<InjVlv_tiETPiI1_mp>"
  cmp_2/1 -> Bitwise_And2/1
  Bitwise_And2/1 -> AndN/2, Scope/2, tws_2/1
  BS_Req/3 -> cmp_3/1, Scope3/1  "<testSig_InjVlv_tiETPoI2_mp>"
  BS_Result/3 -> cmp_3/2, Scope3/2  "<InjVlv_tiETPoI2_mp>"
  cmp_3/1 -> Bitwise_And3/1
  Bitwise_And3/1 -> AndN/3, Scope/3, tws_3/1
  BS_Req/4 -> cmp_4/1, Scope4/1  "<testSig_InjCrv_tiPoI2Pse_mp>"
  BS_Result/4 -> cmp_4/2, Scope4/2  "<InjCrv_tiPoI2Pse_mp>"
  cmp_4/1 -> Bitwise_And4/1
  Bitwise_And4/1 -> AndN/4, Scope/4, tws_4/1
  BS_Req/5 -> cmp_5/1, Scope5/1  "<testSig_InjCrv_tiPiIPse_mp>"
  BS_Result/5 -> cmp_5/2, Scope5/2  "<InjCrv_tiPiIPse_mp>"
  cmp_5/1 -> Bitwise_And5/1
  Bitwise_And5/1 -> AndN/5, Scope/5, tws_5/1
  BS_Req/6 -> cmp_6/1, Scope6/1  "<testSig_InjCrv_tiMI1ET>"
  BS_Result/6 -> cmp_6/2, Scope6/2  "<InjCrv_tiMI1ET>"
  cmp_6/1 -> Bitwise_And6/1
  Bitwise_And6/1 -> AndN/6, Scope/6, tws_6/1
  BS_Req/7 -> cmp_7/1, Scope7/1  "<testSig_InjCrv_tiPiI1ET_mp>"
  BS_Result/7 -> cmp_7/2, Scope7/2  "<InjCrv_tiPiI1ET_mp>"
  cmp_7/1 -> Bitwise_And7/1
  Bitwise_And7/1 -> AndN/7, Scope/7, tws_7/1
  BS_Req/8 -> cmp_8/1, Scope8/1  "<testSig_InjVlv_tiETPiI2_mp>"
  BS_Result/8 -> cmp_8/2, Scope8/2  "<InjVlv_tiETPiI2_mp>"
  cmp_8/1 -> Bitwise_And8/1
  Bitwise_And8/1 -> AndN/8, Scope/8, tws_8/1
  BS_Req/9 -> cmp_9/1, Scope9/1  "<testSig_InjCrv_tiPiI2ET_mp>"
  BS_Result/9 -> cmp_9/2, Scope9/2  "<InjCrv_tiPiI2ET_mp>"
  cmp_9/1 -> Bitwise_And9/1
  Bitwise_And9/1 -> AndN/9, Scope/9, tws_9/1

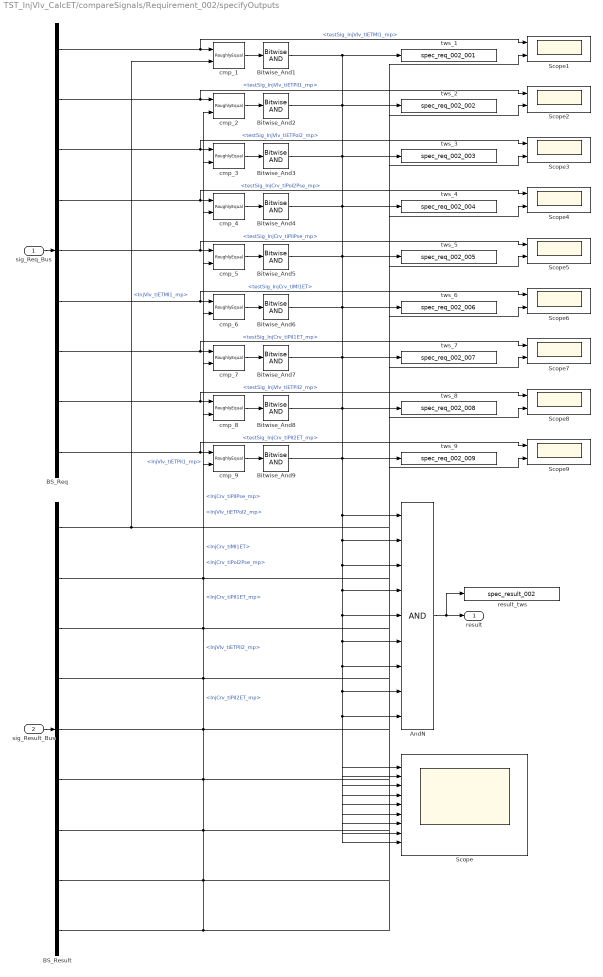
== system TST_InjVlv_CalcET/compareSignals/Requirement_002/specifyOutputs ==
  sig_Req_Bus : Inport
  sig_Result_Bus : Inport  Port=2
  AndN : Logic  Inputs=9
  BS_Req : BusSelector  OutputSignals=testSig_InjVlv_tiETMI1_mp,testSig_InjVlv_tiETPiI1_mp,testSig_InjVlv_tiETPoI2_mp,testSig_InjCrv_tiPoI2Pse_mp,testSig_InjCrv_tiPiIPse_mp,testSig_InjCrv_tiMI1ET,testSig_InjCrv_tiPiI1ET_mp,testSig_InjVlv_tiETPiI2_mp,testSig_InjCrv_tiPiI2ET_mp
  BS_Result : BusSelector  OutputSignals=InjVlv_tiETMI1_mp,InjVlv_tiETPiI1_mp,InjVlv_tiETPoI2_mp,InjCrv_tiPoI2Pse_mp,InjCrv_tiPiIPse_mp,InjCrv_tiMI1ET,InjCrv_tiPiI1ET_mp,InjVlv_tiETPiI2_mp,InjCrv_tiPiI2ET_mp
  Bitwise_And{1..9} (9 alike) : simulink/Logic and Bit Operations/Bitwise Operator  logicop=AND  UseBitMask=off  BitMask=bin2dec('11011001')  BitMaskRealWorld=Stored Integer
  Scope : Scope  NumInputPorts=9
  Scope{1..9} (9 alike) : Scope  NumInputPorts=2
  cmp_{1..9} (9 alike) : UnitTest_Lib/RoughlyEqual  slope=1
  result_tws : ToWorkspace  VariableName=spec_result_002
  tws_1 : ToWorkspace  VariableName=spec_req_002_001
  tws_2 : ToWorkspace  VariableName=spec_req_002_002
  tws_3 : ToWorkspace  VariableName=spec_req_002_003
  tws_4 : ToWorkspace  VariableName=spec_req_002_004
  tws_5 : ToWorkspace  VariableName=spec_req_002_005
  tws_6 : ToWorkspace  VariableName=spec_req_002_006
  tws_7 : ToWorkspace  VariableName=spec_req_002_007
  tws_8 : ToWorkspace  VariableName=spec_req_002_008
  tws_9 : ToWorkspace  VariableName=spec_req_002_009
  result : Outport
  wires:
  sig_Req_Bus/1 -> BS_Req/1
  sig_Result_Bus/1 -> BS_Result/1
  AndN/1 -> result/1, result_tws/1
  BS_Req/1 -> cmp_1/1, Scope1/1  "<testSig_InjVlv_tiETMI1_mp>"
  BS_Result/1 -> cmp_1/2, Scope1/2  "<InjVlv_tiETMI1_mp>"
  cmp_1/1 -> Bitwise_And1/1
  Bitwise_And1/1 -> AndN/1, Scope/1, tws_1/1
  BS_Req/2 -> cmp_2/1, Scope2/1  "<testSig_InjVlv_tiETPiI1_mp>"
  BS_Result/2 -> cmp_2/2, Scope2/2  "<InjVlv_tiETPiI1_mp>"
  cmp_2/1 -> Bitwise_And2/1
  Bitwise_And2/1 -> AndN/2, Scope/2, tws_2/1
  BS_Req/3 -> cmp_3/1, Scope3/1  "<testSig_InjVlv_tiETPoI2_mp>"
  BS_Result/3 -> cmp_3/2, Scope3/2  "<InjVlv_tiETPoI2_mp>"
  cmp_3/1 -> Bitwise_And3/1
  Bitwise_And3/1 -> AndN/3, Scope/3, tws_3/1
  BS_Req/4 -> cmp_4/1, Scope4/1  "<testSig_InjCrv_tiPoI2Pse_mp>"
  BS_Result/4 -> cmp_4/2, Scope4/2  "<InjCrv_tiPoI2Pse_mp>"
  cmp_4/1 -> Bitwise_And4/1
  Bitwise_And4/1 -> AndN/4, Scope/4, tws_4/1
  BS_Req/5 -> cmp_5/1, Scope5/1  "<testSig_InjCrv_tiPiIPse_mp>"
  BS_Result/5 -> cmp_5/2, Scope5/2  "<InjCrv_tiPiIPse_mp>"
  cmp_5/1 -> Bitwise_And5/1
  Bitwise_And5/1 -> AndN/5, Scope/5, tws_5/1
  BS_Req/6 -> cmp_6/1, Scope6/1  "<testSig_InjCrv_tiMI1ET>"
  BS_Result/6 -> cmp_6/2, Scope6/2  "<InjCrv_tiMI1ET>"
  cmp_6/1 -> Bitwise_And6/1
  Bitwise_And6/1 -> AndN/6, Scope/6, tws_6/1
  BS_Req/7 -> cmp_7/1, Scope7/1  "<testSig_InjCrv_tiPiI1ET_mp>"
  BS_Result/7 -> cmp_7/2, Scope7/2  "<InjCrv_tiPiI1ET_mp>"
  cmp_7/1 -> Bitwise_And7/1
  Bitwise_And7/1 -> AndN/7, Scope/7, tws_7/1
  BS_Req/8 -> cmp_8/1, Scope8/1  "<testSig_InjVlv_tiETPiI2_mp>"
  BS_Result/8 -> cmp_8/2, Scope8/2  "<InjVlv_tiETPiI2_mp>"
  cmp_8/1 -> Bitwise_And8/1
  Bitwise_And8/1 -> AndN/8, Scope/8, tws_8/1
  BS_Req/9 -> cmp_9/1, Scope9/1  "<testSig_InjCrv_tiPiI2ET_mp>"
  BS_Result/9 -> cmp_9/2, Scope9/2  "<InjCrv_tiPiI2ET_mp>"
  cmp_9/1 -> Bitwise_And9/1
  Bitwise_And9/1 -> AndN/9, Scope/9, tws_9/1
